simulink model "SpaceRobot"  (R2025b)
settings: Solver=FixedStepAuto  StartTime=0.0  StopTime=100  FixedStep=.01  RelTol=1e-3
libraries: nesl_utility x30, sm_lib x14
settings Model: Creator=gianni  LastModifiedBy=gianni

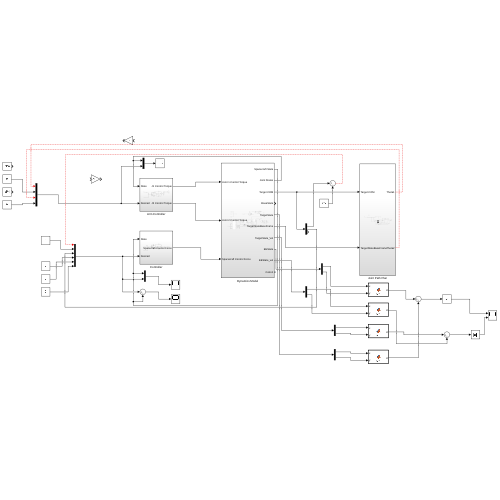
[thumbnail: Simulink's stored preview of the top-level diagram]
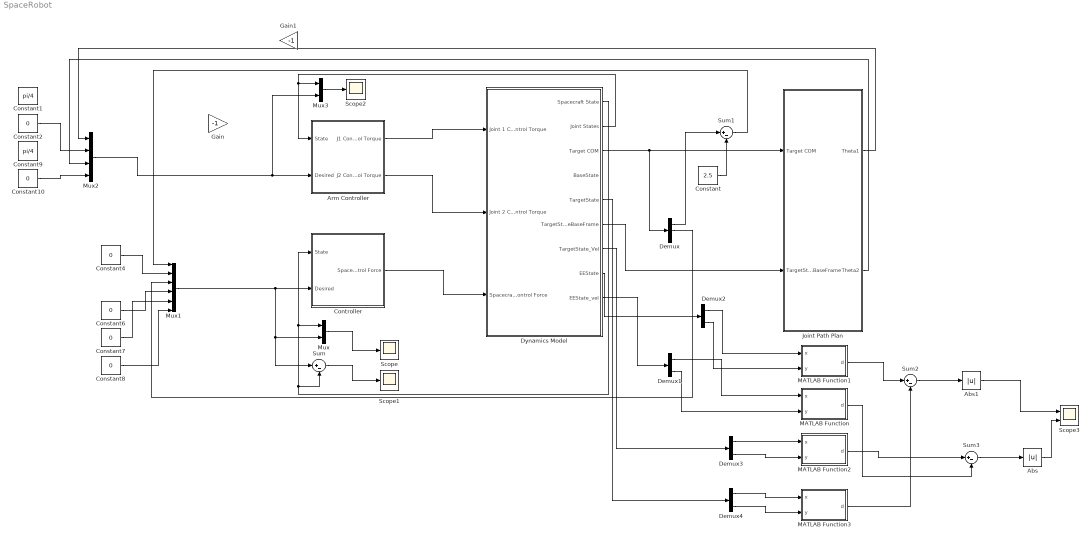
== system SpaceRobot ==
  Abs : Abs  SaturateOnIntegerOverflow=off
  Abs1 : Abs  SaturateOnIntegerOverflow=off
  Arm Controller : Subsystem
  Constant : Constant  Value=2.5
  Constant1 : Constant  Value=pi/4
  Constant{2,4,6..8,10} (6 alike) : Constant  Value=0
  Constant9 : Constant  Value=pi/4
  Controller : Subsystem
  Demux : Demux  Outputs=3
  Demux{1..4} (4 alike) : Demux  Outputs=2
  Dynamics Model : Subsystem
  Gain : Gain  Gain=-1
  Gain1 : Gain  Gain=-1
  Joint Path Plan : Subsystem
  MATLAB Function : MATLAB Function  TreatAsAtomicUnit=on
  MATLAB Function1 : MATLAB Function  TreatAsAtomicUnit=on
  MATLAB Function2 : MATLAB Function  TreatAsAtomicUnit=on
  MATLAB Function3 : MATLAB Function  TreatAsAtomicUnit=on
  Mux : Mux  Inputs=2
  Mux1 : Mux  Inputs=6
  Mux2 : Mux
  Mux3 : Mux  Inputs=2
  Scope : Scope
      settings: ActiveDisplayYMinimum=3.1137212028081822  ActiveDisplayYMaximum=3.1326315046316795
  Scope1 : Scope
      settings: ActiveDisplayYMinimum=-2.5064389373778742  ActiveDisplayYMaximum=3.3179919075778139
  Scope2 : Scope
      settings: ActiveDisplayYMinimum=0.09539230902988971  ActiveDisplayYMaximum=1.6231066757901811  DataLoggingVariableName=ScopeData2
  Scope3 : Scope  NumInputPorts=2
      settings: ActiveDisplayYMinimum=-0.031665709919259558  ActiveDisplayYMaximum=0.066819994550005549  DataLoggingVariableName=ScopeData3
  Sum{,1..3} (4 alike) : Sum  Inputs=|+-
  wires:
  Arm Controller/1(J1 Control Torque) -> Dynamics Model/1(Joint 1 Control Torque)
  Constant4/1 -> Mux1/2
  Sum1/1 -> Mux1/1
  Mux1/1 -> Mux/2, Sum/1, Controller/2(Desired)
  Constant6/1 -> Mux1/4
  Constant7/1 -> Mux1/5
  Constant8/1 -> Mux1/6
  Controller/1(Spacecraft Control Force) -> Dynamics Model/3(Spacecraft Control Force)
  Dynamics Model/1(Spacecraft State) -> Controller/1(State), Mux/1, Sum/2
  Mux/1 -> Scope/1
  Sum/1 -> Scope1/1
  Constant10/1 -> Mux2/4
  Constant2/1 -> Mux2/2
  Mux2/1 -> Mux3/2, Arm Controller/2(Desired)
  Dynamics Model/2(Joint States) -> Arm Controller/1(State), Mux3/1
  Arm Controller/2(J2 Control Torque) -> Dynamics Model/2(Joint 2 Control Torque)
  Mux3/1 -> Scope2/1
  Dynamics Model/3(Target COM) -> Demux/1, Joint Path Plan/1(Target COM)
  Demux/1 -> Sum1/1
  Constant/1 -> Sum1/2
  Demux/2 -> Mux1/3
  Joint Path Plan/1(Theta1) -> Mux2/1
  Joint Path Plan/2(Theta2) -> Mux2/3
  Dynamics Model/6(TargetStateBaseFrame) -> Joint Path Plan/2(TargetStateBaseFrame)
  Dynamics Model/9(EEState_vel) -> Demux1/1
  Demux1/1 -> MATLAB Function/1(x)
  Demux1/2 -> MATLAB Function/2(y)
  Dynamics Model/8(EEState) -> Demux2/1
  Demux2/1 -> MATLAB Function1/1(x)
  Demux2/2 -> MATLAB Function1/2(y)
  Dynamics Model/7(TargetState_Vel) -> Demux3/1
  Demux3/1 -> MATLAB Function2/1(x)
  Demux3/2 -> MATLAB Function2/2(y)
  Dynamics Model/5(TargetState) -> Demux4/1
  Demux4/1 -> MATLAB Function3/1(x)
  Demux4/2 -> MATLAB Function3/2(y)
  MATLAB Function1/1(d) -> Sum2/1
  MATLAB Function3/1(d) -> Sum2/2
  MATLAB Function2/1(d) -> Sum3/1
  MATLAB Function/1(d) -> Sum3/2
  Sum2/1 -> Abs1/1
  Sum3/1 -> Abs/1
  Abs/1 -> Scope3/2
  Abs1/1 -> Scope3/1

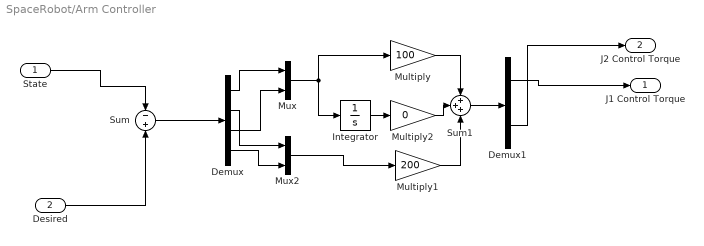
== system SpaceRobot/Arm Controller ==
  State : Inport
  Desired : Inport  Port=2
  Demux : Demux
  Demux1 : Demux  Outputs=2
  Integrator : Integrator
  Multiply : Gain  Gain=100
  Multiply1 : Gain  Gain=200
  Multiply2 : Gain  Gain=0
  Mux : Mux  Inputs=2
  Mux2 : Mux  Inputs=2
  Sum : Sum  Inputs=-+
  Sum1 : Sum  Inputs=+++
  J1 Control Torque : Outport
  J2 Control Torque : Outport  Port=2
  wires:
  Multiply2/1 -> Sum1/2
  Integrator/1 -> Multiply2/1
  Multiply1/1 -> Sum1/3
  Multiply/1 -> Sum1/1
  Mux2/1 -> Multiply1/1
  Mux/1 -> Integrator/1, Multiply/1
  Demux/4 -> Mux2/2
  Demux/2 -> Mux2/1
  Demux/3 -> Mux/2
  Demux/1 -> Mux/1
  Sum/1 -> Demux/1
  Desired/1 -> Sum/2
  State/1 -> Sum/1
  Sum1/1 -> Demux1/1
  Demux1/2 -> J2 Control Torque/1
  Demux1/1 -> J1 Control Torque/1

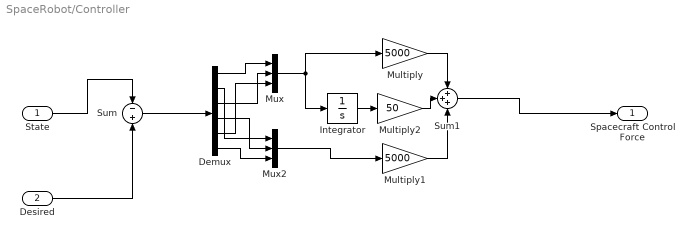
== system SpaceRobot/Controller ==
  State : Inport
  Desired : Inport  Port=2
  Demux : Demux  Outputs=6
  Integrator : Integrator
  Multiply : Gain  Gain=5000
  Multiply1 : Gain  Gain=5000
  Multiply2 : Gain  Gain=50
  Mux : Mux  Inputs=3
  Mux2 : Mux  Inputs=3
  Sum : Sum  Inputs=-+
  Sum1 : Sum  Inputs=+++
  Spacecraft Control Force : Outport
  wires:
  State/1 -> Sum/1
  Desired/1 -> Sum/2
  Sum/1 -> Demux/1
  Demux/1 -> Mux/1
  Demux/3 -> Mux/2
  Demux/5 -> Mux/3
  Demux/2 -> Mux2/1
  Demux/4 -> Mux2/2
  Demux/6 -> Mux2/3
  Mux/1 -> Multiply/1, Integrator/1
  Mux2/1 -> Multiply1/1
  Multiply/1 -> Sum1/1
  Multiply1/1 -> Sum1/3
  Sum1/1 -> Spacecraft Control Force/1
  Integrator/1 -> Multiply2/1
  Multiply2/1 -> Sum1/2

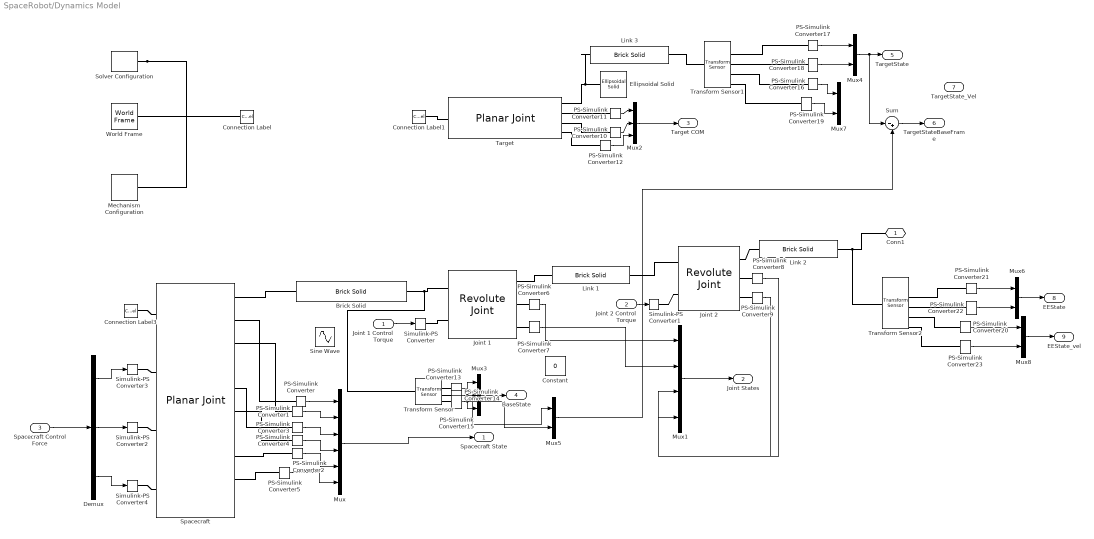
== system SpaceRobot/Dynamics Model ==
  Joint 1 Control Torque : Inport
  Joint 2 Control Torque : Inport  Port=2
  Spacecraft Control Force : Inport  Port=3
  Brick Solid : sm_lib/Body Elements/Brick Solid  BrickDimensions=[2 1 0.01]  BrickDimensionsUnits=m  ExportEntireGeometry=off  InertiaType=CalculateFromGeometry  BasedOnType=Mass  Density=1000  DensityUnits=kg/m^3  Mass=500  MassUnits=kg  CenterOfMass=[0 0 0]  CenterOfMassUnits=m  MomentsOfInertia=[1 1 1]  MomentsOfInertiaUnits=kg*m^2  ProductsOfInertia=[0 0 0]  ProductsOfInertiaUnits=kg*m^2  GraphicType=FromGeometry  MarkerShape=Sphere  MarkerSize=10  GraphicVisPropType=SimpleVisualProperties  GraphicDiffuseColor=[0.5 0.5 0.5]  GraphicOpacity=1  GraphicSpecularColor=[0.5 0.5 0.5 1.0]  GraphicAmbientColor=[0.15 0.15 0.15 1.0]  GraphicEmissiveColor=[0.0 0.0 0.0 1.0]  GraphicShininess=75  DoExposeReferenceFrame=off  SerializedFrames=|
      | <Frames>
      | 
      |   <Frame>
      |     <Id>Frame1</Id>
      |     <Value>
      |       <Name>COM</Name>
      |       <Origin>
      |         <Source>CenterOfMassFrame</Source>
      |         <FeatureName></FeatureName>
      |       </Origin>
      |       <PrimaryAxis>
      |         <DefinedDirection>+Z</DefinedDirection>
      |         <Source>ReferenceFrame</Source>
      |         <SourceDirection>+Z</SourceDirection>
      |         <FeatureName></FeatureName>
      |       </PrimaryAxis>
      |       <SecondaryAxis>
      |         <DefinedDirection>+X</DefinedDirection>
      |         <Source>ReferenceFrame</Source>
      |         <SourceDirection>+X</SourceDirection>
      |         <FeatureName></FeatureName>
      |       </SecondaryAxis>
      |     </Value>
      |   </Frame>
      | 
      |   <Frame>
      |     <Id>Frame3</Id>
      |     <Value>
      |       <Name>ManipulatorBase</Name>
      |       <Origin>
      |         <Source>GeometricFeature</Source>
      |         <FeatureName>+z +x curve</FeatureName>
      |       </Origin>
      |       <PrimaryAxis>
      |         <DefinedDirection>+Z</DefinedDirection>
      |         <Source>ReferenceFrame</Source>
      |         <SourceDirection>+Z</SourceDirection>
      |         <FeatureName></FeatureName>
      |       </PrimaryAxis>
      |       <SecondaryAxis>
      |         <DefinedDirection>+X</DefinedDirection>
      |         <Source>ReferenceFrame</Source>
      |         <SourceDirection>+X</SourceDirection>
      |         <FeatureName></FeatureName>
      |       </SecondaryAxis>
      |     </Value>
      |   </Frame>
      | 
      | </Frames>
  Connection Label : ConnectionLabel  Label=World
  Connection Label1 : ConnectionLabel  Label=World
  Connection Label3 : ConnectionLabel  Label=World
  Constant : Constant  Value=0
  Demux : Demux  Outputs=3
  Ellipsoidal Solid : sm_lib/Body Elements/Ellipsoidal Solid  EllipsoidRadii=[1 .5 .01]  EllipsoidRadiiUnits=m  ExportEntireGeometry=off  InertiaType=CalculateFromGeometry  BasedOnType=Mass  Density=1000  DensityUnits=kg/m^3  Mass=100  MassUnits=kg  CenterOfMass=[0 0 0]  CenterOfMassUnits=m  MomentsOfInertia=[1 1 1]  MomentsOfInertiaUnits=kg*m^2  ProductsOfInertia=[0 0 0]  ProductsOfInertiaUnits=kg*m^2  GraphicType=FromGeometry  MarkerShape=Sphere  MarkerSize=10  GraphicVisPropType=SimpleVisualProperties  GraphicDiffuseColor=[0.5 0.5 0.5]  GraphicOpacity=1  GraphicSpecularColor=[0.5 0.5 0.5 1.0]  GraphicAmbientColor=[0.15 0.15 0.15 1.0]  GraphicEmissiveColor=[0.0 0.0 0.0 1.0]  GraphicShininess=75  DoExposeReferenceFrame=on  SerializedFrames=<Frames><Frame><Id>Frame1</Id><Value><Name>F1</Name><Origin><Source>ReferenceFrame</Source><FeatureName></FeatureName></Origin><PrimaryAxis><DefinedDirection>+Z</DefinedDirection><Source>ReferenceFrame</Source><SourceDirection>+Z</SourceDirection><FeatureName></FeatureName></PrimaryAxis><SecondaryAxis><DefinedDirection>+X</DefinedDirection><Source>ReferenceFrame</Source><SourceDirection>+X</SourceDirection><FeatureName></FeatureName></SecondaryAxis></Value></Frame></Frames>
  Joint 1 : sm_lib/Joints/Revolute Joint  JointMode=Normal  CompositeWrenchDir=FollowerOnBase  CompositeWrenchFrame=BaseFrame  SenseConstraintForce=off  SenseConstraintTorque=off  SenseTotalForce=off  SenseTotalTorque=off  PositionTargetSpecify=off  PositionTargetPriority=High  PositionTargetValue=10  PositionTargetValueUnits=deg  VelocityTargetSpecify=off  VelocityTargetPriority=High  VelocityTargetValue=10  VelocityTargetValueUnits=deg/s  EquilibriumPosition=0  EquilibriumPositionUnits=deg  SpringStiffness=0  SpringStiffnessUnits=N*m/deg  DampingCoefficient=0  DampingCoefficientUnits=N*m/(deg/s)  LowerLimitSpecify=off  LowerLimitBound=-90  LowerLimitBoundUnits=deg  LowerLimitStiffness=1e4  LowerLimitStiffnessUnits=N*m/deg  LowerLimitDamping=10  LowerLimitDampingUnits=N*m/(deg/s)  LowerLimitTransitionRegionWidth=0.1  LowerLimitTransitionRegionWidthUnits=deg  UpperLimitSpecify=off  UpperLimitBound=90  UpperLimitBoundUnits=deg  UpperLimitStiffness=1e4  UpperLimitStiffnessUnits=N*m/deg  UpperLimitDamping=10  UpperLimitDampingUnits=N*m/(deg/s)  UpperLimitTransitionRegionWidth=0.1  UpperLimitTransitionRegionWidthUnits=deg  TorqueActuationMode=InputTorque  MotionActuationMode=ComputedMotion  SensePosition=on  SenseVelocity=on  SenseAcceleration=off  SenseTorqueForce=off  SenseLowerLimitTorqueForce=off  SenseUpperLimitTorqueForce=off
  Joint 2 : sm_lib/Joints/Revolute Joint  JointMode=Normal  CompositeWrenchDir=FollowerOnBase  CompositeWrenchFrame=BaseFrame  SenseConstraintForce=off  SenseConstraintTorque=off  SenseTotalForce=off  SenseTotalTorque=off  PositionTargetSpecify=on  PositionTargetPriority=High  PositionTargetValue=45  PositionTargetValueUnits=deg  VelocityTargetSpecify=off  VelocityTargetPriority=High  VelocityTargetValue=-10  VelocityTargetValueUnits=deg/s  EquilibriumPosition=0  EquilibriumPositionUnits=deg  SpringStiffness=0  SpringStiffnessUnits=N*m/deg  DampingCoefficient=0  DampingCoefficientUnits=N*m/(deg/s)  LowerLimitSpecify=off  LowerLimitBound=-90  LowerLimitBoundUnits=deg  LowerLimitStiffness=1e4  LowerLimitStiffnessUnits=N*m/deg  LowerLimitDamping=10  LowerLimitDampingUnits=N*m/(deg/s)  LowerLimitTransitionRegionWidth=0.1  LowerLimitTransitionRegionWidthUnits=deg  UpperLimitSpecify=off  UpperLimitBound=90  UpperLimitBoundUnits=deg  UpperLimitStiffness=1e4  UpperLimitStiffnessUnits=N*m/deg  UpperLimitDamping=10  UpperLimitDampingUnits=N*m/(deg/s)  UpperLimitTransitionRegionWidth=0.1  UpperLimitTransitionRegionWidthUnits=deg  TorqueActuationMode=InputTorque  MotionActuationMode=ComputedMotion  SensePosition=on  SenseVelocity=on  SenseAcceleration=off  SenseTorqueForce=off  SenseLowerLimitTorqueForce=off  SenseUpperLimitTorqueForce=off
  Link 1 : sm_lib/Body Elements/Brick Solid  BrickDimensions=[1 .05 0.01]  BrickDimensionsUnits=m  ExportEntireGeometry=off  InertiaType=CalculateFromGeometry  BasedOnType=Mass  Density=1000  DensityUnits=kg/m^3  Mass=20  MassUnits=kg  CenterOfMass=[0 0 0]  CenterOfMassUnits=m  MomentsOfInertia=[1 1 1]  MomentsOfInertiaUnits=kg*m^2  ProductsOfInertia=[0 0 0]  ProductsOfInertiaUnits=kg*m^2  GraphicType=FromGeometry  MarkerShape=Sphere  MarkerSize=10  GraphicVisPropType=SimpleVisualProperties  GraphicDiffuseColor=[1 0 0.01569]  GraphicOpacity=1  GraphicSpecularColor=[0.5 0.5 0.5 1.0]  GraphicAmbientColor=[0.15 0.15 0.15 1.0]  GraphicEmissiveColor=[0.0 0.0 0.0 1.0]  GraphicShininess=75  DoExposeReferenceFrame=off  SerializedFrames=<Frames><Frame><Id>Frame1</Id><Value><Name>LinkBase</Name><Origin><Source>GeometricFeature</Source><FeatureName>+z -x curve</FeatureName></Origin><PrimaryAxis><DefinedDirection>+Z</DefinedDirection><Source>ReferenceFrame</Source><SourceDirection>+Z</SourceDirection><FeatureName></FeatureName></PrimaryAxis><SecondaryAxis><DefinedDirection>+X</DefinedDirection><Source>ReferenceFrame</Source><SourceDirection>+X</SourceDirection><FeatureName></FeatureName></SecondaryAxis></Value></Frame><Frame><Id>Frame2</Id><Value><Name>LinkEnd</Name><Origin><Source>GeometricFeature</Source><FeatureName>+z +x curve</FeatureName></Origin><PrimaryAxis><DefinedDirection>+Z</DefinedDirection><Source>ReferenceFrame</Source><SourceDirection>+Z</SourceDirection><FeatureName></FeatureName></PrimaryAxis><SecondaryAxis><DefinedDirection>+X</DefinedDirection><Source>ReferenceFrame</Source><SourceDirection>+X</SourceDirection><FeatureName></FeatureName></SecondaryAxis></Value></Frame></Frames>
  Link 2 : sm_lib/Body Elements/Brick Solid  BrickDimensions=[1 .05 0.01]  BrickDimensionsUnits=m  ExportEntireGeometry=off  InertiaType=CalculateFromGeometry  BasedOnType=Mass  Density=1000  DensityUnits=kg/m^3  Mass=10  MassUnits=kg  CenterOfMass=[0 0 0]  CenterOfMassUnits=m  MomentsOfInertia=[1 1 1]  MomentsOfInertiaUnits=kg*m^2  ProductsOfInertia=[0 0 0]  ProductsOfInertiaUnits=kg*m^2  GraphicType=FromGeometry  MarkerShape=Sphere  MarkerSize=10  GraphicVisPropType=SimpleVisualProperties  GraphicDiffuseColor=[0.08627 0.01961 1]  GraphicOpacity=1  GraphicSpecularColor=[0.5 0.5 0.5 1.0]  GraphicAmbientColor=[0.15 0.15 0.15 1.0]  GraphicEmissiveColor=[0.0 0.0 0.0 1.0]  GraphicShininess=75  DoExposeReferenceFrame=off  SerializedFrames=<Frames><Frame><Id>Frame1</Id><Value><Name>LinkBase</Name><Origin><Source>GeometricFeature</Source><FeatureName>+z -x curve</FeatureName></Origin><PrimaryAxis><DefinedDirection>+Z</DefinedDirection><Source>ReferenceFrame</Source><SourceDirection>+Z</SourceDirection><FeatureName></FeatureName></PrimaryAxis><SecondaryAxis><DefinedDirection>+X</DefinedDirection><Source>ReferenceFrame</Source><SourceDirection>+X</SourceDirection><FeatureName></FeatureName></SecondaryAxis></Value></Frame><Frame><Id>Frame2</Id><Value><Name>LinkEnd</Name><Origin><Source>GeometricFeature</Source><FeatureName>+z +x curve</FeatureName></Origin><PrimaryAxis><DefinedDirection>+Z</DefinedDirection><Source>ReferenceFrame</Source><SourceDirection>+Z</SourceDirection><FeatureName></FeatureName></PrimaryAxis><SecondaryAxis><DefinedDirection>+X</DefinedDirection><Source>ReferenceFrame</Source><SourceDirection>+X</SourceDirection><FeatureName></FeatureName></SecondaryAxis></Value></Frame></Frames>
  Link 3 : sm_lib/Body Elements/Brick Solid  BrickDimensions=[.01 1 0.01]  BrickDimensionsUnits=m  ExportEntireGeometry=off  InertiaType=PointMass  BasedOnType=Mass  Density=1000  DensityUnits=kg/m^3  Mass=0  MassUnits=kg  CenterOfMass=[0 0 0]  CenterOfMassUnits=m  MomentsOfInertia=[1 1 1]  MomentsOfInertiaUnits=kg*m^2  ProductsOfInertia=[0 0 0]  ProductsOfInertiaUnits=kg*m^2  GraphicType=FromGeometry  MarkerShape=Sphere  MarkerSize=10  GraphicVisPropType=SimpleVisualProperties  GraphicDiffuseColor=[1 0 0.01569]  GraphicOpacity=1  GraphicSpecularColor=[0.5 0.5 0.5 1.0]  GraphicAmbientColor=[0.15 0.15 0.15 1.0]  GraphicEmissiveColor=[0.0 0.0 0.0 1.0]  GraphicShininess=75  DoExposeReferenceFrame=on  SerializedFrames=<Frames><Frame><Id>Frame2</Id><Value><Name>TargetPoint</Name><Origin><Source>GeometricFeature</Source><FeatureName>+y surface</FeatureName></Origin><PrimaryAxis><DefinedDirection>+Z</DefinedDirection><Source>ReferenceFrame</Source><SourceDirection>+Z</SourceDirection><FeatureName></FeatureName></PrimaryAxis><SecondaryAxis><DefinedDirection>+X</DefinedDirection><Source>ReferenceFrame</Source><SourceDirection>+X</SourceDirection><FeatureName></FeatureName></SecondaryAxis></Value></Frame></Frames>
  Mechanism Configuration : sm_lib/Utilities/Mechanism Configuration  UniformGravity=Constant  GravityVector=[0 0 -9.80665]*0  GravityVectorUnits=m/s^2  LinearizationDelta=0.001  JointModeTransitionNonlinearIterations=2
  Mux : Mux  Inputs=6
  Mux1 : Mux
  Mux2 : Mux  Inputs=3
  Mux3 : Mux  Inputs=3
  Mux{4..8} (5 alike) : Mux  Inputs=2
  PS-Simulink Converter{,1..23} (24 alike) : nesl_utility/PS-Simulink Converter  PhysicalDomain=network_engine_domain  SubClassName=ps_output  LeftPortType=input  RightPortType=output  PseudoPeriodic=off  Frequencies=[]  VectorFormat=inherit  Unit=inherit  AffineConversion=off
  Simulink-PS Converter{,1..4} (5 alike) : nesl_utility/Simulink-PS Converter  PhysicalDomain=network_engine_domain  SubClassName=ps_input  LeftPortType=input  RightPortType=output  PseudoPeriodic=off  Frequencies=[]  NoiseDistribution=none  NoiseParameters=[]  Unit=1  AffineConversion=off  FilteringAndDerivatives=provide  SimscapeFilterOrder=1  InputFilterTimeConstant=0.001  UdotUserProvided=0
  Sine Wave : Sin  Amplitude=.5  Frequency=0.1  SampleTime=0
  Solver Configuration : nesl_utility/Solver Configuration  PhysicalDomain=network_engine_domain  SubClassName=solver  LeftPortType=input  RightPortType=generic  Tones=[]  Harmonics=[]  SimulateNoise=off  Profile=off  UseLocalSampling=off  EnableSwitchedLinearOptims=on  FrequencyDomain=off  UseCCode=off  RelTol=0.001  AbsTol=1e-06  MinStep=1e-09  ToWorkspace=off  RevertToSquareIcSolve=off  NumHomotopyIterations=100  PhasorMode=off  PhasorModeNumHarmonics=1  ConsistencySolver=NEWTON_FTOL  IndexReductionMethod=DerivativeReplacement  DoDC=off  ResidualTolerance=1e-09  ConsistencyTolSource=GLOBAL  ConsistencyAbsTol=0.001  ConsistencyRelTol=0.001  ConsistencyTolFactor=0.001  UseLocalSolver=off  LocalSolverChoice=NE_BACKWARD_EULER_ADVANCER  ResolveIndetEquations=on  FunctionEvalNumThread=1  LocalSolverSampleTime=0.001  DoFixedCost=off  MaxNonlinIter=3  MaxModeIter=2  ComputeImpulses=off  ImpulseIterations=2  LinearAlgebra=Sparse  LinearAlgebraNumThread=0  EquationFormulation=NE_TIME_EF  DelaysMemoryBudget=1024  AutomaticFiltering=on  FilteringTimeConstant=0.001  PartitionStorageMethod=AS_NEEDED  PartitionMemoryBudget=1024  PartitionMethod=FAST  MultibodyUseLocalSolver=off  MultibodyLocalSolverChoice=ODE1  MultibodyLocalSolverSampleTime=0.001
  Spacecraft : sm_lib/Joints/Planar Joint  JointMode=Normal  CompositeWrenchDir=FollowerOnBase  CompositeWrenchFrame=BaseFrame  SenseConstraintForce=off  SenseConstraintTorque=off  SenseTotalForce=off  SenseTotalTorque=off  PxPositionTargetSpecify=off  PxPositionTargetPriority=High  PxPositionTargetValue=0  PxPositionTargetValueUnits=m  PxVelocityTargetSpecify=off  PxVelocityTargetPriority=High  PxVelocityTargetValue=0  PxVelocityTargetValueUnits=m/s  PxEquilibriumPosition=0  PxEquilibriumPositionUnits=m  PxSpringStiffness=0  PxSpringStiffnessUnits=N/m  PxDampingCoefficient=0  PxDampingCoefficientUnits=N/(m/s)  PxLowerLimitSpecify=off  PxLowerLimitBound=-1  PxLowerLimitBoundUnits=m  PxLowerLimitStiffness=1e6  PxLowerLimitStiffnessUnits=N/m  PxLowerLimitDamping=1e3  PxLowerLimitDampingUnits=N/(m/s)  PxLowerLimitTransitionRegionWidth=1e-4  PxLowerLimitTransitionRegionWidthUnits=m  PxUpperLimitSpecify=off  PxUpperLimitBound=1  PxUpperLimitBoundUnits=m  PxUpperLimitStiffness=1e6  PxUpperLimitStiffnessUnits=N/m  PxUpperLimitDamping=1e3  PxUpperLimitDampingUnits=N/(m/s)  PxUpperLimitTransitionRegionWidth=1e-4  PxUpperLimitTransitionRegionWidthUnits=m  PxTorqueActuationMode=InputTorque  PxMotionActuationMode=ComputedMotion  PxSensePosition=on  PxSenseVelocity=on  PxSenseAcceleration=on  PxSenseTorqueForce=off  PxSenseLowerLimitTorqueForce=off  PxSenseUpperLimitTorqueForce=off  PyPositionTargetSpecify=off  PyPositionTargetPriority=High  PyPositionTargetValue=0  PyPositionTargetValueUnits=m  PyVelocityTargetSpecify=off  PyVelocityTargetPriority=High  PyVelocityTargetValue=0  PyVelocityTargetValueUnits=m/s  PyEquilibriumPosition=0  PyEquilibriumPositionUnits=m  PySpringStiffness=0  PySpringStiffnessUnits=N/m  PyDampingCoefficient=0  PyDampingCoefficientUnits=N/(m/s)  PyLowerLimitSpecify=off  PyLowerLimitBound=-1  PyLowerLimitBoundUnits=m  PyLowerLimitStiffness=1e6  PyLowerLimitStiffnessUnits=N/m  PyLowerLimitDamping=1e3  PyLowerLimitDampingUnits=N/(m/s)  PyLowerLimitTransitionRegionWidth=1e-4  PyLowerLimitTransitionRegionWidthUnits=m  PyUpperLimitSpecify=off  PyUpperLimitBound=1  PyUpperLimitBoundUnits=m  PyUpperLimitStiffness=1e6  PyUpperLimitStiffnessUnits=N/m  PyUpperLimitDamping=1e3  PyUpperLimitDampingUnits=N/(m/s)  PyUpperLimitTransitionRegionWidth=1e-4  PyUpperLimitTransitionRegionWidthUnits=m  PyTorqueActuationMode=InputTorque  PyMotionActuationMode=ComputedMotion  PySensePosition=on  PySenseVelocity=on  PySenseAcceleration=on  PySenseTorqueForce=off  PySenseLowerLimitTorqueForce=off  PySenseUpperLimitTorqueForce=off  RzPositionTargetSpecify=off  RzPositionTargetPriority=High  RzPositionTargetValue=0  RzPositionTargetValueUnits=deg  RzVelocityTargetSpecify=off  RzVelocityTargetPriority=High  RzVelocityTargetValue=0  RzVelocityTargetValueUnits=deg/s  RzEquilibriumPosition=0  RzEquilibriumPositionUnits=deg  RzSpringStiffness=0  RzSpringStiffnessUnits=N*m/deg  RzDampingCoefficient=0  RzDampingCoefficientUnits=N*m/(deg/s)  RzLowerLimitSpecify=off  RzLowerLimitBound=-90  RzLowerLimitBoundUnits=deg  RzLowerLimitStiffness=1e4  RzLowerLimitStiffnessUnits=N*m/deg  RzLowerLimitDamping=10  RzLowerLimitDampingUnits=N*m/(deg/s)  RzLowerLimitTransitionRegionWidth=0.1  RzLowerLimitTransitionRegionWidthUnits=deg  RzUpperLimitSpecify=off  RzUpperLimitBound=90  RzUpperLimitBoundUnits=deg  RzUpperLimitStiffness=1e4  RzUpperLimitStiffnessUnits=N*m/deg  RzUpperLimitDamping=10  RzUpperLimitDampingUnits=N*m/(deg/s)  RzUpperLimitTransitionRegionWidth=0.1  RzUpperLimitTransitionRegionWidthUnits=deg  RzTorqueActuationMode=InputTorque  RzMotionActuationMode=ComputedMotion  RzSensePosition=on  RzSenseVelocity=on  RzSenseAcceleration=on  RzSenseTorqueForce=off  RzSenseLowerLimitTorqueForce=off  RzSenseUpperLimitTorqueForce=off
  Sum : Sum  Inputs=|-+
  Target : sm_lib/Joints/Planar Joint  JointMode=Normal  CompositeWrenchDir=FollowerOnBase  CompositeWrenchFrame=BaseFrame  SenseConstraintForce=off  SenseConstraintTorque=off  SenseTotalForce=off  SenseTotalTorque=off  PxPositionTargetSpecify=on  PxPositionTargetPriority=High  PxPositionTargetValue=5  PxPositionTargetValueUnits=m  PxVelocityTargetSpecify=on  PxVelocityTargetPriority=High  PxVelocityTargetValue=.02  PxVelocityTargetValueUnits=m/s  PxEquilibriumPosition=0  PxEquilibriumPositionUnits=m  PxSpringStiffness=0  PxSpringStiffnessUnits=N/m  PxDampingCoefficient=0  PxDampingCoefficientUnits=N/(m/s)  PxLowerLimitSpecify=off  PxLowerLimitBound=-1  PxLowerLimitBoundUnits=m  PxLowerLimitStiffness=1e6  PxLowerLimitStiffnessUnits=N/m  PxLowerLimitDamping=1e3  PxLowerLimitDampingUnits=N/(m/s)  PxLowerLimitTransitionRegionWidth=1e-4  PxLowerLimitTransitionRegionWidthUnits=m  PxUpperLimitSpecify=off  PxUpperLimitBound=1  PxUpperLimitBoundUnits=m  PxUpperLimitStiffness=1e6  PxUpperLimitStiffnessUnits=N/m  PxUpperLimitDamping=1e3  PxUpperLimitDampingUnits=N/(m/s)  PxUpperLimitTransitionRegionWidth=1e-4  PxUpperLimitTransitionRegionWidthUnits=m  PxTorqueActuationMode=NoTorque  PxMotionActuationMode=ComputedMotion  PxSensePosition=on  PxSenseVelocity=off  PxSenseAcceleration=off  PxSenseTorqueForce=off  PxSenseLowerLimitTorqueForce=off  PxSenseUpperLimitTorqueForce=off  PyPositionTargetSpecify=on  PyPositionTargetPriority=High  PyPositionTargetValue=0  PyPositionTargetValueUnits=m  PyVelocityTargetSpecify=off  PyVelocityTargetPriority=High  PyVelocityTargetValue=0  PyVelocityTargetValueUnits=m/s  PyEquilibriumPosition=0  PyEquilibriumPositionUnits=m  PySpringStiffness=0  PySpringStiffnessUnits=N/m  PyDampingCoefficient=0  PyDampingCoefficientUnits=N/(m/s)  PyLowerLimitSpecify=off  PyLowerLimitBound=-1  PyLowerLimitBoundUnits=m  PyLowerLimitStiffness=1e6  PyLowerLimitStiffnessUnits=N/m  PyLowerLimitDamping=1e3  PyLowerLimitDampingUnits=N/(m/s)  PyLowerLimitTransitionRegionWidth=1e-4  PyLowerLimitTransitionRegionWidthUnits=m  PyUpperLimitSpecify=off  PyUpperLimitBound=1  PyUpperLimitBoundUnits=m  PyUpperLimitStiffness=1e6  PyUpperLimitStiffnessUnits=N/m  PyUpperLimitDamping=1e3  PyUpperLimitDampingUnits=N/(m/s)  PyUpperLimitTransitionRegionWidth=1e-4  PyUpperLimitTransitionRegionWidthUnits=m  PyTorqueActuationMode=NoTorque  PyMotionActuationMode=ComputedMotion  PySensePosition=on  PySenseVelocity=off  PySenseAcceleration=off  PySenseTorqueForce=off  PySenseLowerLimitTorqueForce=off  PySenseUpperLimitTorqueForce=off  RzPositionTargetSpecify=off  RzPositionTargetPriority=High  RzPositionTargetValue=0  RzPositionTargetValueUnits=deg  RzVelocityTargetSpecify=on  RzVelocityTargetPriority=High  RzVelocityTargetValue=1  RzVelocityTargetValueUnits=deg/s  RzEquilibriumPosition=0  RzEquilibriumPositionUnits=deg  RzSpringStiffness=0  RzSpringStiffnessUnits=N*m/deg  RzDampingCoefficient=0  RzDampingCoefficientUnits=N*m/(deg/s)  RzLowerLimitSpecify=off  RzLowerLimitBound=-90  RzLowerLimitBoundUnits=deg  RzLowerLimitStiffness=1e4  RzLowerLimitStiffnessUnits=N*m/deg  RzLowerLimitDamping=10  RzLowerLimitDampingUnits=N*m/(deg/s)  RzLowerLimitTransitionRegionWidth=0.1  RzLowerLimitTransitionRegionWidthUnits=deg  RzUpperLimitSpecify=off  RzUpperLimitBound=90  RzUpperLimitBoundUnits=deg  RzUpperLimitStiffness=1e4  RzUpperLimitStiffnessUnits=N*m/deg  RzUpperLimitDamping=10  RzUpperLimitDampingUnits=N*m/(deg/s)  RzUpperLimitTransitionRegionWidth=0.1  RzUpperLimitTransitionRegionWidthUnits=deg  RzTorqueActuationMode=NoTorque  RzMotionActuationMode=ComputedMotion  RzSensePosition=on  RzSenseVelocity=off  RzSenseAcceleration=off  RzSenseTorqueForce=off  RzSenseLowerLimitTorqueForce=off  RzSenseUpperLimitTorqueForce=off
  Transform Sensor : sm_lib/Frames and Transforms/Transform Sensor  MeasurementFrame=World  RotationSequence=XYZ  SenseAngle=on  SenseAxis=off  SenseQ=off  SenseR=off  SenseRotationSequence=off  SenseOmegaX=off  SenseOmegaY=off  SenseOmegaZ=off  SenseOmega=off  SenseQDot=off  SenseRDot=off  SenseRotationSequenceDot=off  SenseAlphaX=off  SenseAlphaY=off  SenseAlphaZ=off  SenseAlpha=off  SenseQDDot=off  SenseRDDot=off  SenseX=on  SenseY=on  SenseZ=off  SenseXYZ=off  SenseRad=off  SenseAzim=off  SenseDist=off  SenseInc=off  SenseXDot=off  SenseYDot=off  SenseZDot=off  SenseXYZDot=off  SenseRadDot=off  SenseAzimDot=off  SenseDistDot=off  SenseIncDot=off  SenseXDDot=off  SenseYDDot=off  SenseZDDot=off  SenseXYZDDot=off  SenseRadDDot=off  SenseAzimDDot=off  SenseDistDDot=off  SenseIncDDot=off
  Transform Sensor1 : sm_lib/Frames and Transforms/Transform Sensor  MeasurementFrame=World  RotationSequence=XYZ  SenseAngle=off  SenseAxis=off  SenseQ=off  SenseR=off  SenseRotationSequence=off  SenseOmegaX=off  SenseOmegaY=off  SenseOmegaZ=off  SenseOmega=off  SenseQDot=off  SenseRDot=off  SenseRotationSequenceDot=off  SenseAlphaX=off  SenseAlphaY=off  SenseAlphaZ=off  SenseAlpha=off  SenseQDDot=off  SenseRDDot=off  SenseX=on  SenseY=on  SenseZ=off  SenseXYZ=off  SenseRad=off  SenseAzim=off  SenseDist=off  SenseInc=off  SenseXDot=on  SenseYDot=on  SenseZDot=off  SenseXYZDot=off  SenseRadDot=off  SenseAzimDot=off  SenseDistDot=off  SenseIncDot=off  SenseXDDot=off  SenseYDDot=off  SenseZDDot=off  SenseXYZDDot=off  SenseRadDDot=off  SenseAzimDDot=off  SenseDistDDot=off  SenseIncDDot=off
  Transform Sensor2 : sm_lib/Frames and Transforms/Transform Sensor  MeasurementFrame=World  RotationSequence=XYZ  SenseAngle=on  SenseAxis=off  SenseQ=off  SenseR=off  SenseRotationSequence=off  SenseOmegaX=off  SenseOmegaY=off  SenseOmegaZ=off  SenseOmega=off  SenseQDot=off  SenseRDot=off  SenseRotationSequenceDot=off  SenseAlphaX=off  SenseAlphaY=off  SenseAlphaZ=off  SenseAlpha=off  SenseQDDot=off  SenseRDDot=off  SenseX=on  SenseY=on  SenseZ=off  SenseXYZ=off  SenseRad=off  SenseAzim=off  SenseDist=off  SenseInc=off  SenseXDot=on  SenseYDot=on  SenseZDot=off  SenseXYZDot=off  SenseRadDot=off  SenseAzimDot=off  SenseDistDot=off  SenseIncDot=off  SenseXDDot=off  SenseYDDot=off  SenseZDDot=off  SenseXYZDDot=off  SenseRadDDot=off  SenseAzimDDot=off  SenseDistDDot=off  SenseIncDDot=off
  World Frame : sm_lib/Frames and Transforms/World Frame
  Conn1 : PMIOPort  Side=Right
  Spacecraft State : Outport
  Joint States : Outport  Port=2
  Target COM : Outport  Port=3
  BaseState : Outport  Port=4
  TargetState : Outport  Port=5
  TargetStateBaseFrame : Outport  Port=6
  TargetState_Vel : Outport  Port=7
  EEState : Outport  Port=8
  EEState_vel : Outport  Port=9
  wires:
  Demux/2 -> Simulink-PS Converter2/1
  Demux/1 -> Simulink-PS Converter3/1
  Demux/3 -> Simulink-PS Converter4/1
  Mux/1 -> Spacecraft State/1
  Spacecraft Control Force/1 -> Demux/1
  PS-Simulink Converter/1 -> Mux/1
  PS-Simulink Converter1/1 -> Mux/2
  PS-Simulink Converter3/1 -> Mux/3
  PS-Simulink Converter4/1 -> Mux/4
  PS-Simulink Converter2/1 -> Mux/5
  PS-Simulink Converter5/1 -> Mux/6
  Joint 1 Control Torque/1 -> Simulink-PS Converter/1
  Joint 2 Control Torque/1 -> Simulink-PS Converter1/1
  PS-Simulink Converter6/1 -> Mux1/1
  PS-Simulink Converter7/1 -> Mux1/2
  PS-Simulink Converter8/1 -> Mux1/3
  PS-Simulink Converter9/1 -> Mux1/4
  Mux1/1 -> Joint States/1
  PS-Simulink Converter10/1 -> Mux2/2
  PS-Simulink Converter11/1 -> Mux2/1
  Mux2/1 -> Target COM/1
  PS-Simulink Converter12/1 -> Mux2/3
  PS-Simulink Converter13/1 -> Mux3/1
  PS-Simulink Converter14/1 -> Mux5/1, Mux3/2
  Mux3/1 -> BaseState/1
  Mux4/1 -> Sum/1, TargetState/1
  PS-Simulink Converter17/1 -> Mux4/1
  PS-Simulink Converter18/1 -> Mux4/2
  PS-Simulink Converter15/1 -> Mux5/2, Mux3/3
  Mux5/1 -> Sum/2
  Sum/1 -> TargetStateBaseFrame/1
  PS-Simulink Converter16/1 -> Mux7/1
  PS-Simulink Converter19/1 -> Mux7/2
  PS-Simulink Converter21/1 -> Mux6/1
  PS-Simulink Converter22/1 -> Mux6/2
  Mux6/1 -> EEState/1
  Mux8/1 -> EEState_vel/1
  PS-Simulink Converter23/1 -> Mux8/2
  PS-Simulink Converter20/1 -> Mux8/1
  connections:
  Joint 1/RConn1 -- Link 1/LConn1
  Solver Configuration/RConn1 -- World Frame/RConn1 -- Connection Label/LConn1 -- Mechanism Configuration/RConn1
  Simulink-PS Converter/RConn1 -- Joint 1/LConn2
  Brick Solid/RConn1 -- Transform Sensor/LConn1 -- Joint 1/LConn1
  Link 2/RConn1 -- Transform Sensor2/LConn1 -- Conn1/RConn1
  Link 1/RConn1 -- Joint 2/LConn1
  Link 2/LConn1 -- Joint 2/RConn1
  Connection Label3/LConn1 -- Spacecraft/LConn1
  Simulink-PS Converter1/RConn1 -- Joint 2/LConn2
  Brick Solid/LConn1 -- Spacecraft/RConn1
  Simulink-PS Converter2/RConn1 -- Spacecraft/LConn3
  Simulink-PS Converter3/RConn1 -- Spacecraft/LConn2
  Simulink-PS Converter4/RConn1 -- Spacecraft/LConn4
  Spacecraft/RConn2 -- PS-Simulink Converter/LConn1
  Spacecraft/RConn3 -- PS-Simulink Converter1/LConn1
  Spacecraft/RConn5 -- PS-Simulink Converter3/LConn1
  Spacecraft/RConn6 -- PS-Simulink Converter4/LConn1
  Spacecraft/RConn8 -- PS-Simulink Converter2/LConn1
  Spacecraft/RConn9 -- PS-Simulink Converter5/LConn1
  PS-Simulink Converter6/LConn1 -- Joint 1/RConn2
  PS-Simulink Converter8/LConn1 -- Joint 2/RConn2
  PS-Simulink Converter7/LConn1 -- Joint 1/RConn3
  Joint 2/RConn3 -- PS-Simulink Converter9/LConn1
  Connection Label1/LConn1 -- Target/LConn1
  Target/RConn1 -- Link 3/RConn1 -- Ellipsoidal Solid/RConn1
  Target/RConn2 -- PS-Simulink Converter11/LConn1
  Target/RConn3 -- PS-Simulink Converter10/LConn1
  Target/RConn4 -- PS-Simulink Converter12/LConn1
  PS-Simulink Converter13/LConn1 -- Transform Sensor/RConn2
  PS-Simulink Converter14/LConn1 -- Transform Sensor/RConn3
  Transform Sensor/RConn4 -- PS-Simulink Converter15/LConn1
  Link 3/LConn1 -- Transform Sensor1/LConn1
  Transform Sensor1/RConn2 -- PS-Simulink Converter17/LConn1
  PS-Simulink Converter18/LConn1 -- Transform Sensor1/RConn3
  Transform Sensor1/RConn4 -- PS-Simulink Converter16/LConn1
  Transform Sensor1/RConn5 -- PS-Simulink Converter19/LConn1
  PS-Simulink Converter21/LConn1 -- Transform Sensor2/RConn3
  Transform Sensor2/RConn4 -- PS-Simulink Converter22/LConn1
  Transform Sensor2/RConn5 -- PS-Simulink Converter20/LConn1
  Transform Sensor2/RConn6 -- PS-Simulink Converter23/LConn1

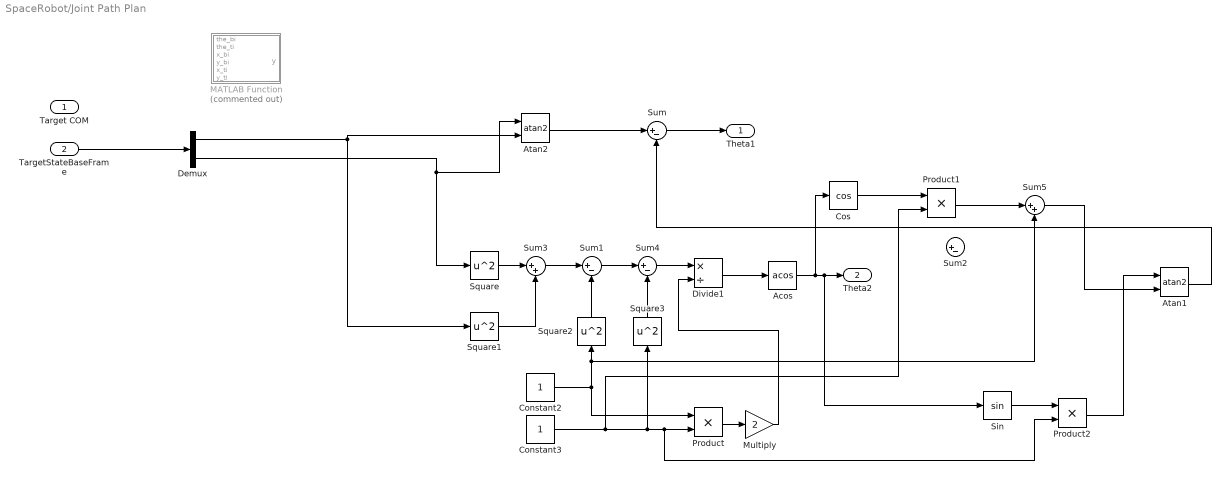
== system SpaceRobot/Joint Path Plan ==
  Target COM : Inport
  TargetStateBaseFrame : Inport  Port=2
  Acos : Trigonometry  Operator=acos
  Atan1 : Trigonometry  Operator=atan2
  Atan2 : Trigonometry  Operator=atan2
  Constant2 : Constant
  Constant3 : Constant
  Cos : Trigonometry  Operator=cos
  Demux : Demux  Outputs=2
  Divide1 : Product  Inputs=*/
  MATLAB Function : MATLAB Function  Commented=on  TreatAsAtomicUnit=on
  Multiply : Gain  Gain=2
  Product : Product
  Product1 : Product
  Product2 : Product
  Sin : Trigonometry
  Square{,1..3} (4 alike) : Math  Operator=square
  Sum{,1..2,4} (4 alike) : Sum  Inputs=|+-
  Sum3 : Sum  Inputs=|++
  Sum5 : Sum  Inputs=|++
  Theta1 : Outport
  Theta2 : Outport  Port=2
  wires:
  Demux/2 -> Square/1, Atan2/1
  Atan2/1 -> Sum/1
  Square1/1 -> Sum3/2
  Square/1 -> Sum3/1
  Sum3/1 -> Sum1/1
  Sum1/1 -> Sum4/1
  Constant2/1 -> Sum5/2, Square2/1, Product/1
  Square2/1 -> Sum1/2
  Square3/1 -> Sum4/2
  Constant3/1 -> Product1/2, Product2/2, Product/2, Square3/1
  Sum4/1 -> Divide1/1
  Multiply/1 -> Divide1/2
  Product/1 -> Multiply/1
  Divide1/1 -> Acos/1
  Acos/1 -> Cos/1, Sin/1, Theta2/1
  Cos/1 -> Product1/1
  Product1/1 -> Sum5/1
  Sin/1 -> Product2/1
  Product2/1 -> Atan1/1
  Sum5/1 -> Atan1/2
  Atan1/1 -> Sum/2
  Sum/1 -> Theta1/1
  TargetStateBaseFrame/1 -> Demux/1
  Demux/1 -> Atan2/2, Square1/1

== matlab function SpaceRobot/MATLAB Function ==
  data: x input; d output; y input
function d = fcn(x,y)
d = sqrt(x^2 + y^2);

== matlab function SpaceRobot/Joint Path Plan/MATLAB Function ==
  data: the_bi input; y output; the_ti input; x_bi input; y_bi input; x_ti input; y_ti input
function y = fcn(the_bi,the_ti,x_bi, y_bi, x_ti,y_ti)
b_0 = 0.5;
the_tb = the_ti-theb_i;
R_tb = [cos(the_tb) sin(the_tb)
        -sin(the_tb) cos(the_tb)];
y_tpi = yti+ b_0*sin(the_ti);
x_tpi = xti+ b_0*cos(the_ti);
p_tb = [x_tpi-x_bi; y_tpi-y_bi];

T_tb = [R_tb p_tb;
     0 0 1];



y = u;

== matlab function SpaceRobot/MATLAB Function1 ==
  data: x input; d output; y input
function d = fcn(x,y)
d = sqrt(x^2 + y^2);

== matlab function SpaceRobot/MATLAB Function2 ==
  data: x input; d output; y input
function d = fcn(x,y)
d = sqrt(x^2 + y^2);

== matlab function SpaceRobot/MATLAB Function3 ==
  data: x input; d output; y input
function d = fcn(x,y)
d = sqrt(x^2 + y^2);
